simulink model "lr_10"  (R2014b)
settings: Solver=ode45  StartTime=0.0  StopTime=20  MaxStep=0.001  RelTol=1e-3
settings Model: Creator=maksimka  LastModifiedBy=maksimka

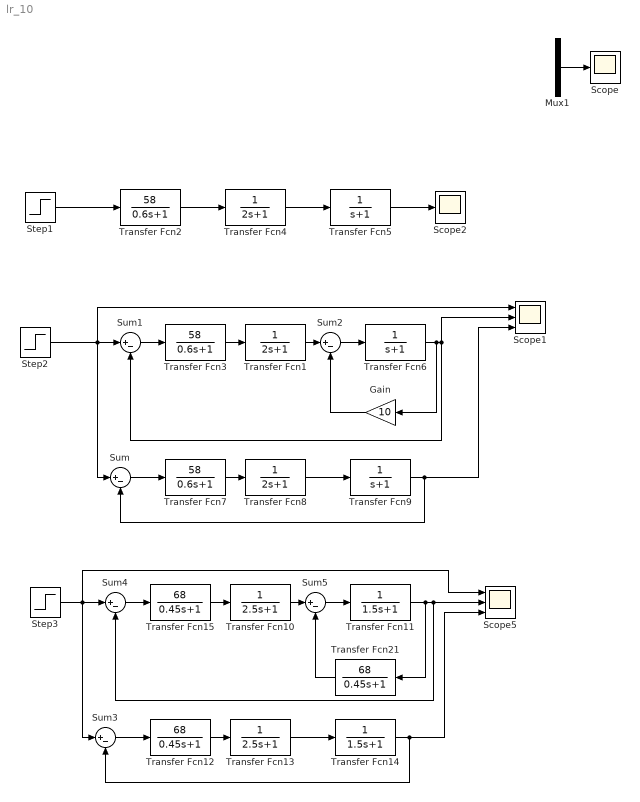
== system lr_10 ==
  Gain : Gain  Gain=10
  Mux1 : Mux  Inputs=2
  Scope : Scope
      settings: TimeRange=20  YMin=-1  YMax=1  MaxDataPoints=50000
  Scope1 : Scope  NumInputPorts=3
      settings: TimeRange=0.03861003861003898  YMin=15~-5~-5  YMax=18.6364~5~5
  Scope2 : Scope
      settings: TimeRange=20  YMin=-1  YMax=1  SaveName=ScopeData2  MaxDataPoints=50000
  Scope5 : Scope  NumInputPorts=3
      settings: TimeRange=0.03861003861003898  YMin=15~-5~-5  YMax=18.6364~5~5  SaveName=ScopeData5
  Step1 : Step  SampleTime=0
  Step2 : Step  Time=0  SampleTime=0
  Step3 : Step  Time=0  SampleTime=0
  Sum{,1..5} (6 alike) : Sum  Inputs=|+-
  Transfer Fcn1 : TransferFcn  Denominator=[2 1]
  Transfer Fcn10 : TransferFcn  Denominator=[2.5 1]
  Transfer Fcn11 : TransferFcn  Denominator=[1.5 1]
  Transfer Fcn12 : TransferFcn  Numerator=[68]  Denominator=[0.45 1]
  Transfer Fcn13 : TransferFcn  Denominator=[2.5 1]
  Transfer Fcn14 : TransferFcn  Denominator=[1.5 1]
  Transfer Fcn15 : TransferFcn  Numerator=[68]  Denominator=[0.45 1]
  Transfer Fcn2 : TransferFcn  Numerator=[58]  Denominator=[0.6 1]
  Transfer Fcn21 : TransferFcn  Numerator=[68]  Denominator=[0.45 1]
  Transfer Fcn3 : TransferFcn  Numerator=[58]  Denominator=[0.6 1]
  Transfer Fcn4 : TransferFcn  Denominator=[2 1]
  Transfer Fcn5 : TransferFcn  Denominator=[1 1]
  Transfer Fcn6 : TransferFcn  Denominator=[1 1]
  Transfer Fcn7 : TransferFcn  Numerator=[58]  Denominator=[0.6 1]
  Transfer Fcn8 : TransferFcn  Denominator=[2 1]
  Transfer Fcn9 : TransferFcn  Denominator=[1 1]
  wires:
  Mux1/1 -> Scope/1
  Step1/1 -> Transfer Fcn2/1
  Transfer Fcn4/1 -> Transfer Fcn5/1
  Transfer Fcn2/1 -> Transfer Fcn4/1
  Transfer Fcn5/1 -> Scope2/1
  Transfer Fcn3/1 -> Transfer Fcn1/1
  Transfer Fcn6/1 -> Scope1/2, Sum1/2, Gain/1
  Sum1/1 -> Transfer Fcn3/1
  Step2/1 -> Scope1/1, Sum/1, Sum1/1
  Transfer Fcn8/1 -> Transfer Fcn9/1
  Transfer Fcn7/1 -> Transfer Fcn8/1
  Sum/1 -> Transfer Fcn7/1
  Transfer Fcn1/1 -> Sum2/1
  Sum2/1 -> Transfer Fcn6/1
  Transfer Fcn9/1 -> Scope1/3, Sum/2
  Gain/1 -> Sum2/2
  Transfer Fcn15/1 -> Transfer Fcn10/1
  Transfer Fcn11/1 -> Transfer Fcn21/1, Scope5/2, Sum4/2
  Sum4/1 -> Transfer Fcn15/1
  Step3/1 -> Scope5/1, Sum3/1, Sum4/1
  Transfer Fcn13/1 -> Transfer Fcn14/1
  Transfer Fcn12/1 -> Transfer Fcn13/1
  Sum3/1 -> Transfer Fcn12/1
  Transfer Fcn10/1 -> Sum5/1
  Sum5/1 -> Transfer Fcn11/1
  Transfer Fcn14/1 -> Scope5/3, Sum3/2
  Transfer Fcn21/1 -> Sum5/2
